simulink model "control_model"  (R2018b)
settings: Solver=VariableStepAuto  StartTime=0.0  StopTime=10.0  RelTol=1e-3
libraries: simulink x2, simulink_extras x1
settings Model: Creator=geraldlow  LastModifiedBy=geraldlow

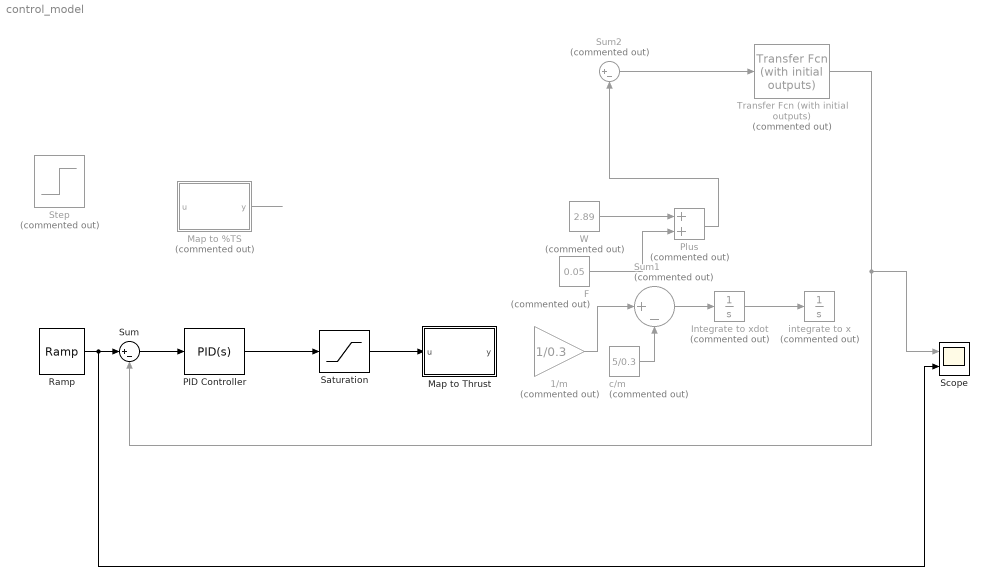
== system control_model ==
  1/m : Gain  Commented=on  Gain=1/0.3
  F : Constant  Commented=on  Value=0.05
  Integrate to xdot : Integrator  Commented=on
  Map to %TS : MATLAB Function  Commented=on  TreatAsAtomicUnit=on
  Map to Thrust : MATLAB Function  TreatAsAtomicUnit=on
  PID Controller : simulink/Continuous/PID Controller  Controller=PID  Form=Parallel  TimeDomain=Continuous-time  SampleTime=-1  IntegratorMethod=Forward Euler  FilterMethod=Forward Euler  ControllerParametersSource=internal  P=0.787889377400751  I=0.0368848665120051  D=4.132620855504  UseFilter=on  N=5.45397025421619  TunerSelectOption=Transfer Function Based (PID Tuner App)  InitialConditionSource=internal  InitialConditionForIntegrator=0  InitialConditionForFilter=0  DifferentiatorICPrevScaledInput=0  ExternalReset=none  TrackingMode=off  Kt=1  LimitOutput=off  UpperSaturationLimit=inf  LowerSaturationLimit=-inf  LinearizeAsGain=on  AntiWindupMode=none  Kb=1  POutMin=[]  POutMax=[]  IOutMin=[]  IOutMax=[]  DOutMin=[]  DOutMax=[]  NOutMin=[]  NOutMax=[]  SumOutMin=[]  SumOutMax=[]  SaturationOutMin=[]  SaturationOutMax=[]  PParamMin=[]  PParamMax=[]  IParamMin=[]  IParamMax=[]  DParamMin=[]  DParamMax=[]  NParamMin=[]  NParamMax=[]  KbParamMin=[]  KbParamMax=[]  KtParamMin=[]  KtParamMax=[]  KbOutMin=[]  KbOutMax=[]  KtOutMin=[]  KtOutMax=[]  IntegratorOutMin=[]  IntegratorOutMax=[]  FilterOutMin=[]  FilterOutMax=[]  SumI1OutMin=[]  SumI1OutMax=[]  SumI2OutMin=[]  SumI2OutMax=[]  SumI3OutMin=[]  SumI3OutMax=[]  SumI4OutMin=[]  SumI4OutMax=[]  SumDOutMin=[]  SumDOutMax=[]  DifferentiatorOutMin=[]  DifferentiatorOutMax=[]  FilterDiffOutCoefMin=[]  FilterDiffOutCoefMax=[]  ReciprocalOutMin=[]  ReciprocalOutMax=[]  SumDenOutMin=[]  SumDenOutMax=[]  SumNumOutMin=[]  SumNumOutMax=[]  DivideOutMin=[]  DivideOutMax=[]  IntegratorContinuousStateAttributes=''  IntegratorStateMustResolveToSignalObject=off  IntegratorRTWStateStorageClass=Auto  FilterContinuousStateAttributes=''  FilterStateMustResolveToSignalObject=off  FilterRTWStateStorageClass=Auto  ParallelPVariant=InternalParameters  IdealPVariant=Disabled  IVariant=InternalParameters  DVariant=InternalParameters  IntegratorVariant=Continuous  SatVariant=Disabled  AWVariant=Passthrough  PCopyVariant=Disabled  TRVariant=Disabled  FdbkBlocksVariant=Forward  IdealPFdbkVariant=Disabled  SatFdbkVariant=Disabled  DerivativeFilterVariant=ContFilter  NVariant=InternalParameters  NCopyVariant=Disabled  FilterICVariant=InternalICsFilter  IntegratorICVariant=InternalICs  ExternalResetVariant=Disabled  TRSumVariant=Passthrough  SumFdbkVariant=Disabled  SumVariant=Sum_PID
  Plus : Sum  Commented=on
  Ramp : simulink/Sources/Ramp  slope=5  start=0  InitialOutput=0
  Saturation : Saturate  UpperLimit=100  LowerLimit=0
  Scope : Scope  NumInputPorts=2
  Step : Step  Commented=on  Time=2  After=5  SampleTime=0
  Sum : Sum  Inputs=|+-
  Sum1 : Sum  Commented=on  Inputs=|+-
  Sum2 : Sum  Commented=on  Inputs=|+-
  Transfer Fcn (with initial outputs) : simulink_extras/Additional Linear/Transfer Fcn (with initial outputs)  Commented=on  N=[1]  D="[0.3  0  0]"  Y0=.5  U0=0
  W : Constant  Commented=on  Value=2.89
  c/m : Constant  Commented=on  Value=5/0.3
  integrate to x : Integrator  Commented=on
  wires:
  Map to %TS/1(y) -> ?
  Sum/1 -> PID Controller/1
  PID Controller/1 -> Saturation/1
  1/m/1 -> Sum1/1
  c/m/1 -> Sum1/2
  Sum1/1 -> Integrate to xdot/1
  Integrate to xdot/1 -> integrate to x/1
  Transfer Fcn (with initial outputs)/1 -> Sum/2, Scope/1
  W/1 -> Plus/1
  Sum2/1 -> Transfer Fcn (with initial outputs)/1
  F/1 -> Plus/2
  Plus/1 -> Sum2/2
  Ramp/1 -> Scope/2, Sum/1
  Saturation/1 -> Map to Thrust/1(u)

== matlab function control_model/Map to Thrust ==
  data: u input; y output
function y = fcn(u)
y = 0.0707*u + 0.393;

== matlab function control_model/Map to %TS ==
  data: u input; y output
function y = fcn(u)

y = u;
